simulink model "wheelModel"  (R2023a)
settings: Solver=VariableStepAuto  StartTime=0.0  StopTime=5  RelTol=1e-3
libraries: fl_lib x15, sdl_lib x5, nesl_utility x4
settings Model: Creator=ashu  LastModifiedBy=ashu
settings OptimizationCC: ReuseModelBlockBuffer=off

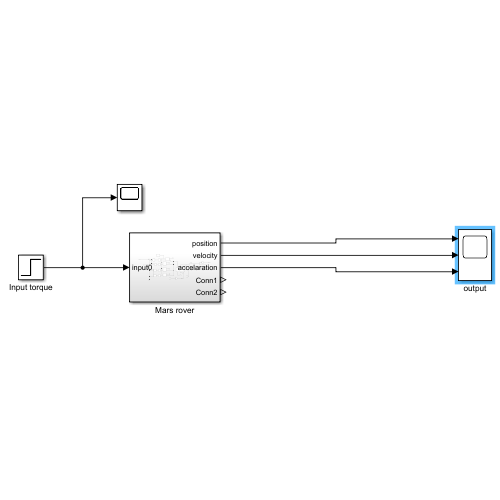
[thumbnail: Simulink's stored preview of the top-level diagram]
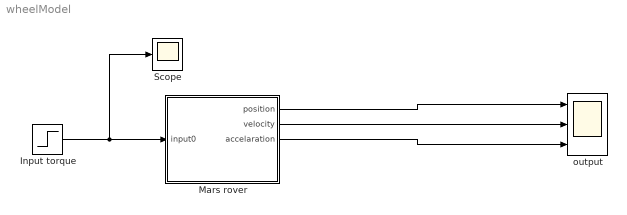
== system wheelModel ==
  Input torque : Step  Time=0  Before=30  After=30  SampleTime=0
  Mars rover : Subsystem
  Scope : Scope
  output : Scope  NumInputPorts=3
  wires:
  Input torque/1 -> Scope/1, Mars rover/1(input0)
  Mars rover/1(position) -> output/1
  Mars rover/2(velocity) -> output/2
  Mars rover/3(accelaration) -> output/3

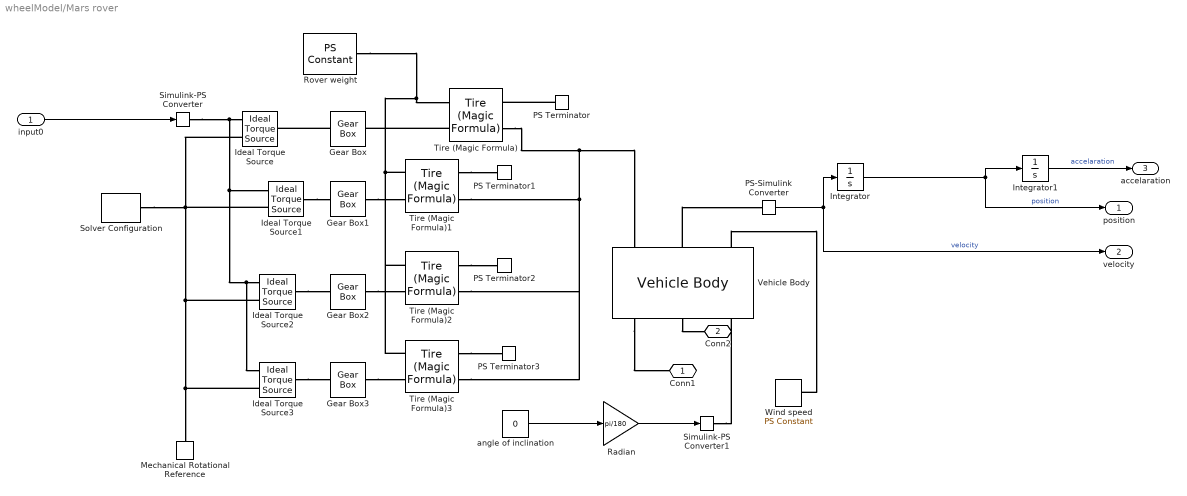
== system wheelModel/Mars rover ==
  input0 : Inport
  Gear Box{,1..3} (4 alike) : fl_lib/Mechanical/Mechanisms/Gear Box  ratio=1  t_in_specify=off  t_in_priority=None  t_in=0 N*m  t_in_nominal_specify=off  t_in_nominal_unit=N*m  t_in_nominal_value=1  t_out_specify=off  t_out_priority=None  t_out=0 N*m  t_out_nominal_specify=off  t_out_nominal_unit=N*m  t_out_nominal_value=1
  Ideal Torque Source{,1..3} (4 alike) : fl_lib/Mechanical/Mechanical Sources/Ideal Torque Source
  Integrator : Integrator
  Integrator1 : Integrator
  Mechanical Rotational Reference : fl_lib/Mechanical/Rotational Elements/Mechanical Rotational Reference
  PS Terminator{,1..3} (4 alike) : fl_lib/Physical Signals/Sinks/PS Terminator
  PS-Simulink Converter : nesl_utility/PS-Simulink Converter  PhysicalDomain=network_engine_domain  SubClassName=ps_output  LeftPortType=input  RightPortType=output  PseudoPeriodic=off  Frequencies=[]  VectorFormat=inherit  Unit=inherit  AffineConversion=off
  Radian : Gain  Gain=pi/180
  Rover weight : fl_lib/Physical Signals/Sources/PS Constant  constant=50*9.81/4 N
  Simulink-PS Converter : nesl_utility/Simulink-PS Converter  PhysicalDomain=network_engine_domain  SubClassName=ps_input  LeftPortType=input  RightPortType=output  PseudoPeriodic=off  Frequencies=[]  NoiseDistribution=none  NoiseParameters=[]  Unit=1  AffineConversion=off  FilteringAndDerivatives=provide  SimscapeFilterOrder=1  InputFilterTimeConstant=0.001  UdotUserProvided=0
  Simulink-PS Converter1 : nesl_utility/Simulink-PS Converter  PhysicalDomain=network_engine_domain  SubClassName=ps_input  LeftPortType=input  RightPortType=output  PseudoPeriodic=off  Frequencies=[]  NoiseDistribution=none  NoiseParameters=[]  Unit=1  AffineConversion=off  FilteringAndDerivatives=provide  SimscapeFilterOrder=1  InputFilterTimeConstant=0.001  UdotUserProvided=0
  Solver Configuration : nesl_utility/Solver Configuration  PhysicalDomain=network_engine_domain  SubClassName=solver  LeftPortType=input  RightPortType=generic  Tones=[]  Harmonics=[]  SimulateNoise=off  Profile=off  UseLocalSampling=off  EnableSwitchedLinearOptims=on  FrequencyDomain=off  UseCCode=off  RelTol=0.001  AbsTol=0.001  MinStep=1e-09  ToWorkspace=off  RevertToSquareIcSolve=off  NumHomotopyIterations=100  PhasorMode=off  PhasorModeNumHarmonics=1  ConsistencySolver=NEWTON_XTOL_AFTER_FTOL  IndexReductionMethod=DerivativeReplacement  DoDC=off  ResidualTolerance=1e-09  ConsistencyTolSource=GLOBAL  ConsistencyAbsTol=0.001  ConsistencyRelTol=0.001  ConsistencyTolFactor=0.001  UseLocalSolver=off  LocalSolverChoice=NE_BACKWARD_EULER_ADVANCER  ResolveIndetEquations=on  FunctionEvalNumThread=1  LocalSolverSampleTime=0.001  DoFixedCost=off  MaxNonlinIter=3  MaxModeIter=2  ComputeImpulses=off  ImpulseIterations=2  LinearAlgebra=auto  LinearAlgebraNumThread=0  EquationFormulation=NE_TIME_EF  DelaysMemoryBudget=1024  AutomaticFiltering=on  FilteringTimeConstant=0.001  PartitionStorageMethod=AS_NEEDED  PartitionMemoryBudget=1024  PartitionMethod=ROBUST
  Tire (Magic Formula){,1..3} (4 alike) : sdl_lib/Tires & Vehicles/Tire (Magic Formula)  parameterization=sdl.enum.magic_tire_model.constant  F_z1=3000 N  F_x1=3500 N  kappa1=10  B_m=12  C_m=2.3  D_m=0.82  E_m=01  fz0=4000 N  p_Cx=1.685  p_Dx=[1.21, -.037]  p_Ex=[.344, .095, -.02, 0]  p_Kx=[21.51, -.163, .245]  p_Hx=[-.002, .002]  p_Vx=[0, 0]  rolling_radius_model=sdl.enum.RollingRadiusParameterization.Constant  r_e=0.15 m  r_0=0.3 m  breff=8.39  dreff=0.26  freff=0.074  q_re0=0.99  q_v1=0.008  longvl=17 m/s  cz=5e5 N/m  model_resistance=simscape.enum.onoff.off  resistance_model=sdl.enum.rollingResistanceParameterization.constant  coeff=0.015  p_tire=250e3 Pa  alpha=-0.003  beta=0.97  coeff_a=84e-4  coeff_b=6.2e-4 s/m  coeff_c=1.6e-4 s^2/m^2  p_tire0=240e3 Pa  fz0_resistance=4000 N  vH0=16 m/s  q_Sy=[.0082, 0, .0014, .001, 0, 0, 1.08, -.5]  v_thr=0.001 m/s  enable_scaling_coefficients=false  lfzO=1  lcx=1  lmux=1  lex=1  lkx=1  lhx=1  lvx=1  lmy=1  model_compliance=sdl.enum.compliance.off  stiffness=1e6 N/m  damping=1000 N*s/m  model_inertia=sdl.enum.model_inertia.on  inertia=1*0.15^2 kg*m^2  initial_velocity=0 rad/s  vxlow=0.1 m/s  v_tr_thr=0.1*(0.1) m/s  kpumin=-1e5  kpumax=1e5
  Vehicle Body : sdl_lib/Tires & Vehicles/Vehicle Body  mass=50 kg  n_w=1  x_f=0.1 m  x_r=0.1 m  y_c=0.1 m  mass_var=simscape.enum.onoff.off  g=9.81 m/s^2  liftoff_warning=simscape.enum.onoff.off  area=1.8 m^2  Cd=2.1  rho=1.293 kg/m^3  model_pitch=simscape.enum.onoff.off  inertia=4000 kg*m^2  suspension_model=sdl.enum.linearTLU.linear  k_f=1e4 N/m  b_f=1e4 N*s/m  k_r=1e4 N/m  b_r=1e4 N*s/m  k_f_TLU=[-2000, -1000, 0, 1000, 2000] N  x_f_TLU=[-.4, -.2, 0, .2, .4] m  b_f_TLU=[-200, -100, 0, 100, 200] N  v_f_TLU=[-4, -2, 0, 2, 4] m/s  k_r_TLU=[-2000, -1000, 0, 1000, 2000] N  x_r_TLU=[-.4, -.2, 0, .2, .4] m  b_r_TLU=[-200, -100, 0, 100, 200] N  v_r_TLU=[-4, -2, 0, 2, 4] m/s  interp_method=simscape.enum.interpolation.linear  extrap_method=simscape.enum.extrapolation.linear  model_hardstop=simscape.enum.onoff.off  upper_bound_f=.25 m  lower_bound_f=-.25 m  stop_k_f=1e6 N/m  stop_b_f=150 N*s/m  upper_bound_r=.25 m  lower_bound_r=-.25 m  stop_k_r=1e6 N/m  stop_b_r=150 N*s/m  initial_pitch=0 rad  initial_pitch_rate=0 rad/s  v_specify=off  v_priority=High  v=2 m/s  v_nominal_specify=off  v_nominal_unit=m/s  v_nominal_value=1
  Wind speed : fl_lib/Physical Signals/Sources/PS Constant  constant=0 m/s
  angle of inclination : Constant  Value=0
  Conn1 : PMIOPort  Side=Right
  Conn2 : PMIOPort  Port=2  Side=Right
  position : Outport
  velocity : Outport  Port=2
  accelaration : Outport  Port=3
  wires:
  angle of inclination/1 -> Radian/1
  PS-Simulink Converter/1 -> velocity/1, Integrator/1  "velocity"
  Radian/1 -> Simulink-PS Converter1/1
  Integrator/1 -> Integrator1/1, position/1  "position"
  input0/1 -> Simulink-PS Converter/1
  Integrator1/1 -> accelaration/1  "accelaration"
  connections:
  Ideal Torque Source/RConn2 -- Solver Configuration/RConn1 -- Ideal Torque Source1/RConn2 -- Ideal Torque Source2/RConn2 -- Ideal Torque Source3/RConn2 -- Mechanical Rotational Reference/LConn1
  Simulink-PS Converter1/RConn1 -- Vehicle Body/RConn3
  Vehicle Body/LConn2 -- PS-Simulink Converter/LConn1
  Ideal Torque Source1/LConn1 -- Gear Box1/LConn1
  Tire (Magic Formula)1/RConn1 -- PS Terminator1/LConn1
  Rover weight/RConn1 -- Tire (Magic Formula)3/LConn1 -- Tire (Magic Formula)2/LConn1 -- Tire (Magic Formula)1/LConn1 -- Tire (Magic Formula)/LConn1
  Gear Box/LConn1 -- Ideal Torque Source/LConn1
  Simulink-PS Converter/RConn1 -- Ideal Torque Source1/RConn1 -- Ideal Torque Source3/RConn1 -- Ideal Torque Source2/RConn1 -- Ideal Torque Source/RConn1
  Gear Box2/RConn1 -- Tire (Magic Formula)2/LConn2
  PS Terminator/LConn1 -- Tire (Magic Formula)/RConn1
  Tire (Magic Formula)/RConn2 -- Tire (Magic Formula)3/RConn2 -- Tire (Magic Formula)2/RConn2 -- Tire (Magic Formula)1/RConn2 -- Vehicle Body/LConn1
  Tire (Magic Formula)/LConn2 -- Gear Box/RConn1
  Ideal Torque Source3/LConn1 -- Gear Box3/LConn1
  Vehicle Body/LConn3 -- Wind speed/RConn1
  Tire (Magic Formula)3/RConn1 -- PS Terminator3/LConn1
  Gear Box1/RConn1 -- Tire (Magic Formula)1/LConn2
  Gear Box3/RConn1 -- Tire (Magic Formula)3/LConn2
  Ideal Torque Source2/LConn1 -- Gear Box2/LConn1
  Tire (Magic Formula)2/RConn1 -- PS Terminator2/LConn1
  Vehicle Body/RConn1 -- Conn1/RConn1
  Vehicle Body/RConn2 -- Conn2/RConn1
